simulink model "planta_ajuste_metodo_rele"  (R2023b)
settings: Solver=ode23t  StartTime=0.0  StopTime=10  MaxStep=T  RelTol=1e-3  EnableMultiTasking=on
undefined symbols (not defined in the file): T
settings Model: Creator=fernandopassold  LastModifiedBy=hmvke
settings SolverCC: AlgebraicLoopSolver=TrustRegion
settings DataIOCC: LimitDataPoints=on  SaveFormat=Array  ReturnWorkspaceOutputs=off
settings OptimizationCC: LifeSpan=inf
settings DebuggingCC: UnconnectedInputMsg=warning  UnconnectedOutputMsg=warning  UnconnectedLineMsg=warning  SFUnexpectedBacktrackingDiag=warning  SFNoUnconditionalDefaultTransitionDiag=warning  SFExecutionAtInitializationDiag=none  ArithmeticOperatorsInVariantConditions=warning
settings HardwareCC: ProdBitPerPointer=32  ProdBitPerSizeT=32  ProdBitPerPtrDiffT=32  ProdLargestAtomicFloat=None  ProdIntDivRoundTo=Undefined  ProdEndianess=Unspecified  ProdWordSize=32  ProdHWDeviceType=32-bit Generic
settings ModelReferenceCC: EnableRefExpFcnMdlSchedulingChecks=on  PropagateSignalLabelsOutOfModel=off
settings SFSimCC: SimUseLocalCustomCode=off  CustomCodeUndefinedFunction=UseInterfaceOnly
settings RTWCC: RTWUseLocalCustomCode=off
settings CodeAppCC: StateflowObjectComments=on
settings GRTTargetCC: TargetLangStandard=C89/C90 (ANSI)
settings ConfigComp: CovMetricSettings=dw  CovSaveCumulativeToWorkspaceVar=on  CovSaveSingleToWorkspaceVar=on  CovExternalEMLEnable=off

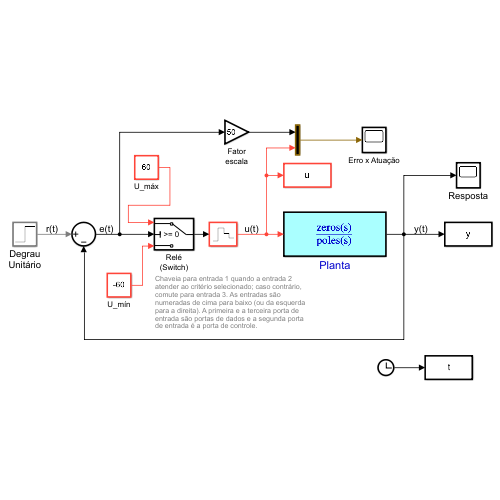
[thumbnail: Simulink's stored preview of the top-level diagram]
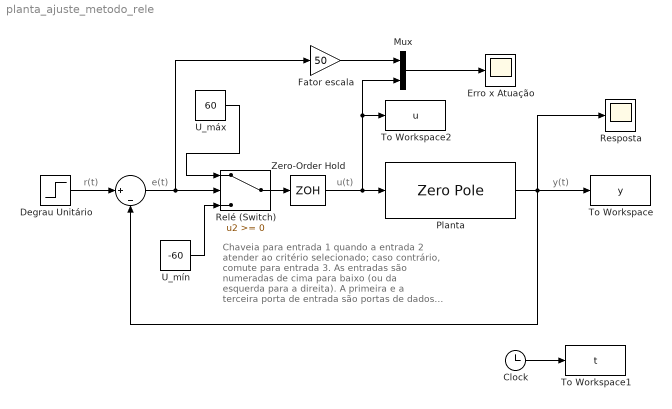
== system planta_ajuste_metodo_rele ==
  note: Chaveia para entrada 1 quando a entrada 2 atender ao critério selecionado; caso contrário, comute para entrada 3. As entradas são numeradas de cima para baixo (ou da esquerda para a direita). A primeira e a terceira porta de entrada são portas de dados e a segunda porta de entrada é a porta de controle.
  note: r(t)
  note: e(t)
  note: u(t)
  note: y(t)
  " " : Sum  Inputs=||+|-
  Clock : Clock
  Degrau Unitário : Step  SampleTime=0
  Erro x Atuação : Scope
  Fator escala : Gain  Gain=50
  Mux : Mux  Inputs=2
  Planta : ZeroPole  Zeros=[ ]  Poles="[-1  -2   -10]"
  Relé (Switch) : Switch  SaturateOnIntegerOverflow=off  InputSameDT=off
  Resposta : Scope
  To Workspace : ToWorkspace  VariableName=y  SaveFormat=Timeseries  SampleTime=-1
  To Workspace1 : ToWorkspace  VariableName=t  SampleTime=-1
  To Workspace2 : ToWorkspace  VariableName=u  SaveFormat=Timeseries  SampleTime=T
  U_máx : Constant  Value=60  SampleTime=T
  U_mín : Constant  Value=-60  SampleTime=T
  Zero-Order Hold : ZeroOrderHold  SampleTime=T
  wires:
  Degrau Unitário/1 -> " "/1
  Zero-Order Hold/1 -> Mux/2, To Workspace2/1, Planta/1
  Planta/1 -> " "/2, Resposta/1, To Workspace/1
  Clock/1 -> To Workspace1/1
  " "/1 -> Fator escala/1, Relé (Switch)/2
  Mux/1 -> Erro x Atuação/1
  Relé (Switch)/1 -> Zero-Order Hold/1
  U_máx/1 -> Relé (Switch)/1
  U_mín/1 -> Relé (Switch)/3
  Fator escala/1 -> Mux/1
